simulink model "Position_sensor"  (R2022b)
settings: Solver=VariableStepAuto  StartTime=0.0  StopTime=10.0  RelTol=1e-3
libraries: simulink x2
settings Model: Creator=Dell  LastModifiedBy=Dell

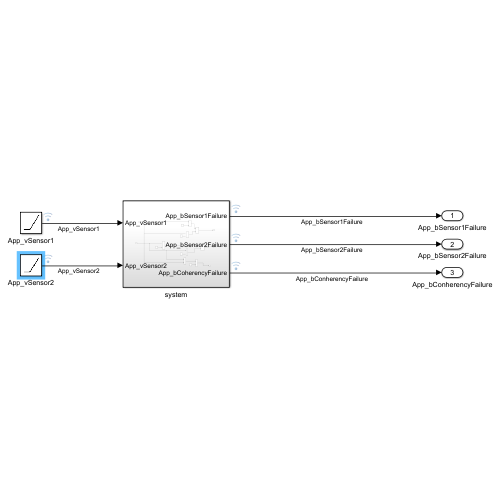
[thumbnail: Simulink's stored preview of the top-level diagram]
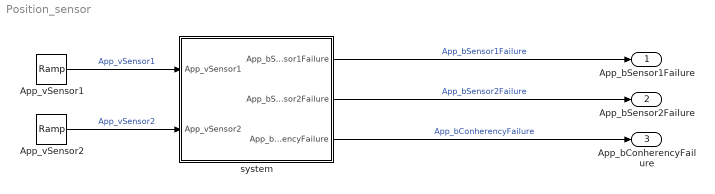
== system Position_sensor ==
  App_vSensor1 : simulink/Sources/Ramp  slope=0.4  start=0  InitialOutput=0.5
  App_vSensor2 : simulink/Sources/Ramp  slope=-0.4  start=0  InitialOutput=4.5
  system : Subsystem
  App_bSensor1Failure : Outport
  App_bSensor2Failure : Outport  Port=2
  App_bConherencyFailure : Outport  Port=3
  wires:
  App_vSensor1/1 -> system/1(App_vSensor1)  "App_vSensor1"
  App_vSensor2/1 -> system/2(App_vSensor2)  "App_vSensor2"
  system/1(App_bSensor1Failure) -> App_bSensor1Failure/1  "App_bSensor1Failure"
  system/2(App_bSensor2Failure) -> App_bSensor2Failure/1  "App_bSensor2Failure"
  system/3(App_bCoherencyFailure) -> App_bConherencyFailure/1  "App_bConherencyFailure"

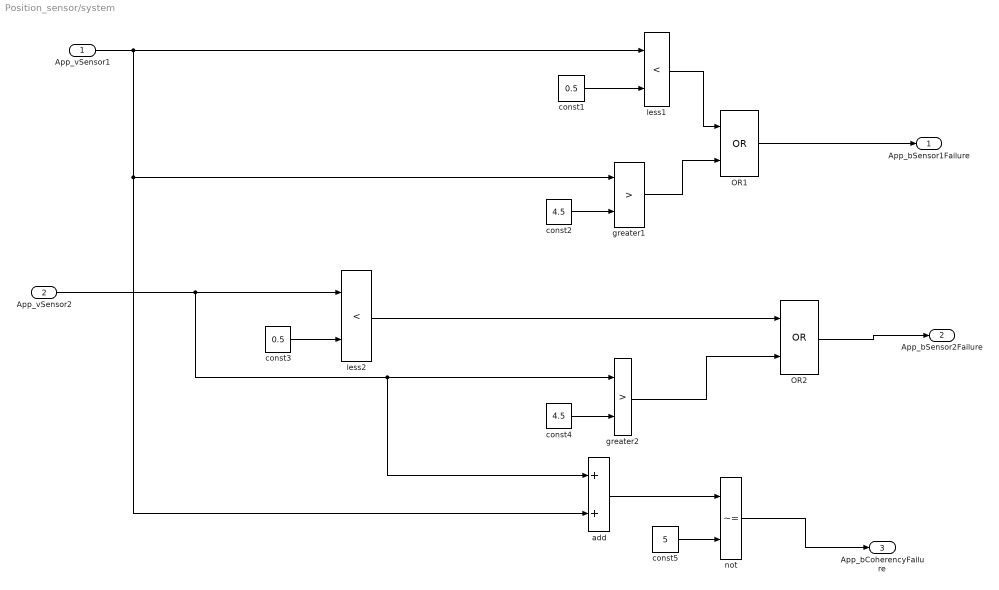
== system Position_sensor/system ==
  App_vSensor1 : Inport
  App_vSensor2 : Inport  Port=2
  OR1 : Logic  Operator=OR  AllPortsSameDT=off  OutDataTypeStr=boolean
  OR2 : Logic  Operator=OR  AllPortsSameDT=off  OutDataTypeStr=boolean
  add : Sum
  const1 : Constant  Value=0.5
  const2 : Constant  Value=4.5
  const3 : Constant  Value=0.5
  const4 : Constant  Value=4.5
  const5 : Constant  Value=5
  greater1 : RelationalOperator  Operator=>  OutDataTypeStr=boolean  RndMeth=Simplest  InputSameDT=off
  greater2 : RelationalOperator  Operator=>  OutDataTypeStr=boolean  RndMeth=Simplest  InputSameDT=off
  less1 : RelationalOperator  Operator=<  OutDataTypeStr=boolean  RndMeth=Simplest  InputSameDT=off
  less2 : RelationalOperator  Operator=<  OutDataTypeStr=boolean  RndMeth=Simplest  InputSameDT=off
  not : RelationalOperator  Operator=~=  OutDataTypeStr=boolean  RndMeth=Simplest  InputSameDT=off
  App_bSensor1Failure : Outport
  App_bSensor2Failure : Outport  Port=2
  App_bCoherencyFailure : Outport  Port=3
  wires:
  App_vSensor1/1 -> less1/1, add/2, greater1/1
  const1/1 -> less1/2
  const2/1 -> greater1/2
  less1/1 -> OR1/1
  greater1/1 -> OR1/2
  OR1/1 -> App_bSensor1Failure/1
  App_vSensor2/1 -> add/1, greater2/1, less2/1
  const3/1 -> less2/2
  const4/1 -> greater2/2
  less2/1 -> OR2/1
  greater2/1 -> OR2/2
  OR2/1 -> App_bSensor2Failure/1
  add/1 -> not/1
  const5/1 -> not/2
  not/1 -> App_bCoherencyFailure/1
